simulink library "Power_FuelCell1Motor"  (R2019b)
settings: Solver=VariableStepAuto  StartTime=0.0  StopTime=10.0  RelTol=1e-3
undefined symbols (not defined in the file or in its folder): Init, Powertrain
libraries: fl_lib x84, nesl_utility x29, GasN_lib x21, SimscapeFluids_lib x6, simulink_extras x5, customMath_lib x5, ee_lib x3, gn_supplement_lib x2, simulink x2, custom_dcdc_uni_lib x1, sm_lib x1
(part 2 of 2)

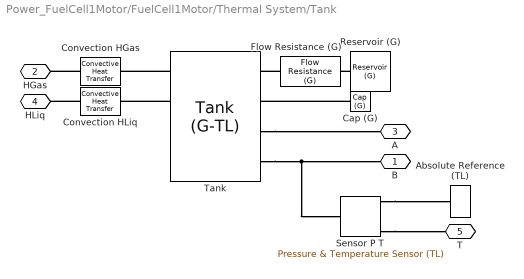
== system Power_FuelCell1Motor/FuelCell1Motor/Thermal System/Tank ==
  Absolute Reference (TL) : fl_lib/Thermal Liquid/Elements/Absolute Reference (TL)
      settings: SourceProductName=Simscape  SourceProductBaseCode=SS
  Cap (G) : fl_lib/Gas/Elements/Cap (G)  p_specify=off  p_priority=None  p=0.101325 MPa  p_nominal_specify=off  p_nominal_unit=MPa  p_nominal_value=1  T_specify=off  T_priority=None  T=293.15 K  T_nominal_specify=off  T_nominal_unit=K  T_nominal_value=1
      settings: SourceProductName=Simscape  SourceProductBaseCode=SS
  Convection HGas : fl_lib/Thermal/Thermal Elements/Convective Heat Transfer  area=1e-2 m^2  heat_tr_coeff=20 W/(m^2 * K)  T_specify=off  T_priority=None  T=0 K  T_nominal_specify=off  T_nominal_unit=K  T_nominal_value=1  Q_specify=off  Q_priority=None  Q=0 W  Q_nominal_specify=off  Q_nominal_unit=W  Q_nominal_value=1
  Convection HLiq : fl_lib/Thermal/Thermal Elements/Convective Heat Transfer  area=1e-4 m^2  heat_tr_coeff=20 W/(m^2 * K)  T_specify=off  T_priority=None  T=0 K  T_nominal_specify=off  T_nominal_unit=K  T_nominal_value=1  Q_specify=off  Q_priority=None  Q=0 W  Q_nominal_specify=off  Q_nominal_unit=W  Q_nominal_value=1
  Flow Resistance (G) : fl_lib/Gas/Elements/Flow Resistance (G)  delta_p_nominal=0.001 MPa  mdot_nominal=0.1 kg/s  rho_nominal=0 kg/m^3  area=0.01 m^2  laminar_fraction=1e-3
      settings: SourceProductName=Simscape  SourceProductBaseCode=SS  InternalSimscapePortConfiguration="{\"Bottom\":[],\"Left\":[{\"id\":\"A\",\"label\":\"A\",\"type\":\"foundation.gas.gas\"}],\"Right\":[{\"id\":\"B\",\"label\":\"B\",\"type\":\"foundation.gas.gas\"}],\"Top\":[]}"
  Reservoir (G) : fl_lib/Gas/Elements/Reservoir (G)  pressure_spec=1  reservoir_pressure=0.101325 MPa  reservoir_temperature=25 degC  area_A=0.001 m^2
      settings: SourceProductName=Simscape  SourceProductBaseCode=SS
  Sensor P T : fl_lib/Thermal Liquid/Sensors/Pressure & Temperature Sensor (TL)
      settings: SourceProductName=Simscape  SourceProductBaseCode=SS  InternalSimscapePortConfiguration="{\"Bottom\":[],\"Left\":[{\"id\":\"A\",\"label\":\"A\",\"type\":\"foundation.thermal_liquid.thermal_liquid\"}],\"Right\":[{\"id\":\"B\",\"label\":\"B\",\"type\":\"foundation.thermal_liquid.thermal_liquid\"},{\"id\":\"P\",\"label\":\"P\",\"type\":\"output\"},{\"id\":\"T\",\"label\":\"T\",\"type\":\"output\"}],\"Top\":[]}"
  Tank : SimscapeFluids_lib/Fluid Network Interfaces/Tanks & Accumulators/Tank (G-TL)  volume_total=Cooling.Tank.volume.Value m^3  volume_spec=1  tank_area=Cooling.Tank.area.Value m^2  level_TLU=[0, 3, 5] m  volume_TLU=[0, 4, 6] m^3  inlet_height=0.01 m  inlet_areas_A1B1=Cooling.Tank.areaA1B1.Value m^2  area_A2=0.01^2*pi m^2  g=9.81 m/s^2  p_gas_tank_specify=off  p_gas_tank_priority=High  p_gas_tank=0.101325 MPa  p_gas_tank_nominal_specify=off  p_gas_tank_nominal_unit=MPa  p_gas_tank_nominal_value=1  T_gas_tank_specify=on  T_gas_tank_priority=High  T_gas_tank=Cooling.Tank.TgasInit.Value K  T_gas_tank_nominal_specify=off  T_gas_tank_nominal_unit=K  T_gas_tank_nominal_value=1  rho_gas_tank_specify=off  rho_gas_tank_priority=None  rho_gas_tank=1.2 kg/m^3  rho_gas_tank_nominal_specify=off  rho_gas_tank_nominal_unit=kg/m^3  rho_gas_tank_nominal_value=1  T_liquid_tank_specify=on  T_liquid_tank_priority=High  T_liquid_tank=Cooling.Tank.TliquidInit.Value K  T_liquid_tank_nominal_specify=off  T_liquid_tank_nominal_unit=K  T_liquid_tank_nominal_value=1  level_specify=on  level_priority=High  level="Cooling.Tank.heightInit.Value  m"  level_nominal_specify=off  level_nominal_unit=m  level_nominal_value=1  volume_liquid_specify=off  volume_liquid_priority=None  volume_liquid=5 m^3  volume_liquid_nominal_specify=off  volume_liquid_nominal_unit=m^3  volume_liquid_nominal_value=1  mass_liquid_specify=off  mass_liquid_priority=None  mass_liquid=5e+3 kg  mass_liquid_nominal_specify=off  mass_liquid_nominal_unit=kg  mass_liquid_nominal_value=1  inlet_heights_A2B2=Cooling.Tank.heightA2B2.Value m  inlet_areas_A2B2=Cooling.Tank.areaA2B2.Value m^2  inlet_heights_A2B2C2=[.1, .05, 0] m  inlet_areas_A2B2C2=[.01, .01, .01] m^2
      settings: SourceProductName=Simscape Fluids  SourceProductBaseCode=SH  InternalSimscapePortConfiguration="{\"Bottom\":[],\"Left\":[{\"id\":\"A1\",\"label\":\"A1\",\"type\":\"foundation.gas.gas\"},{\"id\":\"B1\",\"label\":\"B1\",\"type\":\"foundation.gas.gas\"},{\"id\":\"A2\",\"label\":\"A2\",\"type\":\"foundation.thermal_liquid.thermal_liquid\"},{\"id\":\"B2\",\"label\":\"B2\",\"type\":\"foundation.thermal_liquid.thermal_liquid\"}],\"Right\":[{\"id\":\"H1\",\"label\":\"H1\",\"type\":\"foundation.thermal.thermal\"},{\"id\":\"H2\",\"label\":\"H2\",\"type\":\"foundation.thermal.thermal\"},{\"id\":\"V_out\",\"label\":\"V\",\"type\":\"output\"},{\"id\":\"L_out\",\"label\":\"L\",\"type\":\"output\"}],\"Top\":[]}"
  B : PMIOPort  Side=Left
  HGas : PMIOPort  Port=2  Side=Left
  A : PMIOPort  Port=3  Side=Right
  HLiq : PMIOPort  Port=4  Side=Left
  T : PMIOPort  Port=5  Side=Right
  connections:
  Flow Resistance (G)/RConn1 -- Tank/LConn1
  Tank/LConn3 -- A/RConn1
  Tank/RConn2 -- Convection HLiq/LConn1
  Reservoir (G)/LConn1 -- Flow Resistance (G)/LConn1
  Convection HGas/RConn1 -- HGas/RConn1
  Cap (G)/LConn1 -- Tank/LConn2
  Tank/LConn4 -- Sensor P T/LConn1 -- B/RConn1
  Sensor P T/RConn1 -- Absolute Reference (TL)/LConn1
  Sensor P T/RConn3 -- T/RConn1
  Convection HLiq/RConn1 -- HLiq/RConn1
  Tank/RConn1 -- Convection HGas/LConn1

== system Power_FuelCell1Motor/FuelCell1Motor/Thermal System/Thermal Circuit Converter FC ==
  Conductive Heat Transfer : fl_lib/Thermal/Thermal Elements/Conductive Heat Transfer  area=Cooling.Converter.conductionArea.Value m^2  thickness=Cooling.Converter.conductionThickness.Value m  th_cond=Cooling.Converter.conductivity.Value W/(m*K)  T_specify=off  T_priority=None  T=0 K  T_nominal_specify=off  T_nominal_unit=K  T_nominal_value=1  Q_specify=off  Q_priority=None  Q=0 W  Q_nominal_specify=off  Q_nominal_unit=W  Q_nominal_value=1
      settings: SourceProductName=Simscape
  Thermal Mass : fl_lib/Thermal/Thermal Elements/Thermal Mass  mass=Cooling.Converter.mThermal.Value kg  sp_heat=Cooling.Converter.Cp.Value J/kg/K  T_specify=off  T_priority=High  T=300 K  T_nominal_specify=off  T_nominal_unit=K  T_nominal_value=1  Q_specify=off  Q_priority=None  Q=0 W  Q_nominal_specify=off  Q_nominal_unit=W  Q_nominal_value=1
  A : PMIOPort  Side=Left
  B : PMIOPort  Port=2  Side=Right
  connections:
  Conductive Heat Transfer/RConn1 -- Thermal Mass/LConn1 -- B/RConn1
  Conductive Heat Transfer/LConn1 -- A/RConn1

== system Power_FuelCell1Motor/FuelCell1Motor/Thermal System/Thermal Circuit MotorF ==
  Case-Ambient Insulated : fl_lib/Thermal/Thermal Elements/Perfect Insulator  T_specify=off  T_priority=None  T=0 K  T_nominal_specify=off  T_nominal_unit=K  T_nominal_value=1
      settings: SourceProductName=Simscape
  Iron Stack-Case Conductance : fl_lib/Thermal/Thermal Elements/Conductive Heat Transfer  area=Cooling.MotorF.statorArea.Value cm^2  thickness=Cooling.MotorF.statorThickness.Value cm  th_cond=Cooling.MotorF.statorConductivity.Value W/(m*K)  T_specify=off  T_priority=None  T=0 K  T_nominal_specify=off  T_nominal_unit=K  T_nominal_value=1  Q_specify=off  Q_priority=None  Q=0 W  Q_nominal_specify=off  Q_nominal_unit=W  Q_nominal_value=1
      settings: SourceProductName=Simscape
  Motor Case Thermal Mass : fl_lib/Thermal/Thermal Elements/Thermal Mass  mass=Cooling.MotorF.statormThermal.Value kg  sp_heat="Cooling.MotorF.statorCp.Value  J/kg/K"  T_specify=off  T_priority=High  T=300 K  T_nominal_specify=off  T_nominal_unit=K  T_nominal_value=1  Q_specify=off  Q_priority=None  Q=0 W  Q_nominal_specify=off  Q_nominal_unit=W  Q_nominal_value=1
  Stator Iron Thermal Mass : fl_lib/Thermal/Thermal Elements/Thermal Mass  mass=Cooling.MotorF.w2smThermal.Value kg  sp_heat=Cooling.MotorF.w2sCp.Value J/kg/K  T_specify=off  T_priority=High  T=300 K  T_nominal_specify=off  T_nominal_unit=K  T_nominal_value=1  Q_specify=off  Q_priority=None  Q=0 W  Q_nominal_specify=off  Q_nominal_unit=W  Q_nominal_value=1
  Winding Conductance : fl_lib/Thermal/Thermal Elements/Conductive Heat Transfer  area=Cooling.MotorF.windingArea.Value cm^2  thickness=Cooling.MotorF.windingThickness.Value cm  th_cond=Cooling.MotorF.windingConductivity.Value W/(m*K)  T_specify=off  T_priority=None  T=0 K  T_nominal_specify=off  T_nominal_unit=K  T_nominal_value=1  Q_specify=off  Q_priority=None  Q=0 W  Q_nominal_specify=off  Q_nominal_unit=W  Q_nominal_value=1
      settings: SourceProductName=Simscape
  Winding Thermal Mass : fl_lib/Thermal/Thermal Elements/Thermal Mass  mass=Cooling.MotorF.windingmThermal.Value kg  sp_heat=Cooling.MotorF.Cp.Value J/kg/K  T_specify=off  T_priority=High  T=300 K  T_nominal_specify=off  T_nominal_unit=K  T_nominal_value=1  Q_specify=off  Q_priority=None  Q=0 W  Q_nominal_specify=off  Q_nominal_unit=W  Q_nominal_value=1
  Winding-Iron Conductance : fl_lib/Thermal/Thermal Elements/Conductive Heat Transfer  area=Cooling.MotorF.w2sArea.Value cm^2  thickness=Cooling.MotorF.w2sThickness.Value cm  th_cond=Cooling.MotorF.w2sConductivity.Value W/(m*K)  T_specify=off  T_priority=None  T=0 K  T_nominal_specify=off  T_nominal_unit=K  T_nominal_value=1  Q_specify=off  Q_priority=None  Q=0 W  Q_nominal_specify=off  Q_nominal_unit=W  Q_nominal_value=1
      settings: SourceProductName=Simscape
  A : PMIOPort  Side=Left
  B : PMIOPort  Port=2  Side=Right
  connections:
  Winding Conductance/RConn1 -- A/RConn1
  B/RConn1 -- Winding-Iron Conductance/LConn1 -- Iron Stack-Case Conductance/LConn1 -- Stator Iron Thermal Mass/LConn1
  Case-Ambient Insulated/LConn1 -- Iron Stack-Case Conductance/RConn1 -- Motor Case Thermal Mass/LConn1
  Winding Thermal Mass/LConn1 -- Winding-Iron Conductance/RConn1 -- Winding Conductance/LConn1

== system Power_FuelCell1Motor/FuelCell1Motor/Fuel Cell/Fuel Cell/Cap ==
  Absolute Reference (N Gas) : GasN_lib/Absolute Reference (N Gas)
      settings: InternalSimscapePortConfiguration="{\"Bottom\":[],\"Left\":[{\"id\":\"A\",\"label\":\"\",\"type\":\"GasN.GasN\"}],\"Right\":[],\"Top\":[]}"
  Sensor P T : GasN_lib/Pressure and Temperature Sensor (N Gas)
      settings: InternalSimscapePortConfiguration="{\"Bottom\":[],\"Left\":[{\"id\":\"A\",\"label\":\"A\",\"type\":\"GasN.GasN\"}],\"Right\":[{\"id\":\"p\",\"label\":\"p\",\"type\":\"output\"},{\"id\":\"T\",\"label\":\"T\",\"type\":\"output\"},{\"id\":\"B\",\"label\":\"B\",\"type\":\"GasN.GasN\"}],\"Top\":[]}"
  A : PMIOPort  Side=Left
  connections:
  Sensor P T/LConn1 -- A/RConn1
  Absolute Reference (N Gas)/LConn1 -- Sensor P T/RConn3

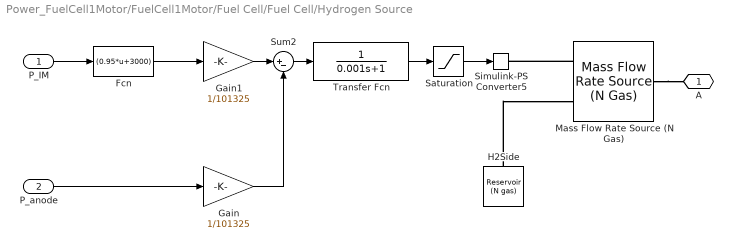
== system Power_FuelCell1Motor/FuelCell1Motor/Fuel Cell/Fuel Cell/Hydrogen Source ==
  P_IM : Inport
  P_anode : Inport  Port=2
  Fcn : Fcn  Expr=(0.95*u+3000)
  Gain : Gain  Gain=1/101325
  Gain1 : Gain  Gain=1/101325
  H2Side : GasN_lib/Reservoir (N gas)  p0=FuelCell.AnodeReservoir.p.Value MPa  T0=FuelCell.AnodeReservoir.T.Value degC  constCond=true  comp=GasN.composition_enum.mole  y0=FuelCell.AnodeReservoir.rMoleFractions.Value'  x0=[1; 0; 0; 0]  area=FuelCell.AnodeReservoir.areaPort.Value cm^2
      settings: InternalSimscapePortConfiguration="{\"Bottom\":[],\"Left\":[{\"id\":\"A\",\"label\":\"A\",\"type\":\"GasN.GasN\"}],\"Right\":[],\"Top\":[]}"
  Mass Flow Rate Source (N Gas) : GasN_lib/Mass Flow Rate Source (N Gas)  const_flow=false  flow_rate=0 kg/s  power_spec=foundation.enum.power_spec.none  area_A=FuelCell.Anode.areaPort.Value cm^2  area_B=FuelCell.Anode.areaPort.Value cm^2  mdot_A_specify=off  mdot_A_priority=None  mdot_A=0.1 kg/s  mdot_A_nominal_specify=off  mdot_A_nominal_unit=kg/s  mdot_A_nominal_value=1  mdot_B_specify=off  mdot_B_priority=None  mdot_B=0.1 kg/s  mdot_B_nominal_specify=off  mdot_B_nominal_unit=kg/s  mdot_B_nominal_value=1  phi_A_specify=off  phi_A_priority=None  phi_A=0 J/s  phi_A_nominal_specify=off  phi_A_nominal_unit=J/s  phi_A_nominal_value=1  phi_B_specify=off  phi_B_priority=None  phi_B=0 J/s  phi_B_nominal_specify=off  phi_B_nominal_unit=J/s  phi_B_nominal_value=1  mdot_A_i_specify=off  mdot_A_i_priority=None  mdot_A_i=[ 0; 0; 0; 0 ] kg/s  mdot_A_i_nominal_specify=off  mdot_A_i_nominal_unit=kg/s  mdot_A_i_nominal_value=1  mdot_B_i_specify=off  mdot_B_i_priority=None  mdot_B_i=[ 0; 0; 0; 0 ] kg/s  mdot_B_i_nominal_specify=off  mdot_B_i_nominal_unit=kg/s  mdot_B_i_nominal_value=1
      settings: InternalSimscapePortConfiguration="{\"Bottom\":[],\"Left\":[{\"id\":\"M\",\"label\":\"M\",\"type\":\"input\"},{\"id\":\"A\",\"label\":\"A\",\"type\":\"GasN.GasN\"}],\"Right\":[{\"id\":\"B\",\"label\":\"B\",\"type\":\"GasN.GasN\"}],\"Top\":[]}"
  Saturation : Saturate  UpperLimit=.1  LowerLimit=0.000001  ZeroCross=off
  Simulink-PS Converter5 : nesl_utility/Simulink-PS Converter  PhysicalDomain=network_engine_domain  SubClassName=ps_input  LeftPortType=input  RightPortType=output  PseudoPeriodic=off  Frequencies=[]  NoiseDistribution=none  NoiseParameters=[]  Unit=kg/s  AffineConversion=off  FilteringAndDerivatives=provide  SimscapeFilterOrder=1  InputFilterTimeConstant=0.001  UdotUserProvided=0
  Sum2 : Sum  Inputs=|+-  SaturateOnIntegerOverflow=on  InputSameDT=on  OutDataTypeStr=Inherit: Same as first input
  Transfer Fcn : TransferFcn  Denominator=[0.001 1]
  A : PMIOPort  Side=Right
  wires:
  Transfer Fcn/1 -> Saturation/1
  Gain1/1 -> Sum2/1
  Fcn/1 -> Gain1/1
  Saturation/1 -> Simulink-PS Converter5/1
  Gain/1 -> Sum2/2
  Sum2/1 -> Transfer Fcn/1
  P_IM/1 -> Fcn/1
  P_anode/1 -> Gain/1
  connections:
  Mass Flow Rate Source (N Gas)/LConn1 -- Simulink-PS Converter5/RConn1
  Mass Flow Rate Source (N Gas)/RConn1 -- A/RConn1
  H2Side/LConn1 -- Mass Flow Rate Source (N Gas)/LConn2

== system Power_FuelCell1Motor/FuelCell1Motor/Fuel Cell/Fuel Cell/Oxygen Source ==
  Icmd : Inport
  Chiller : Subsystem
  Compressor : Subsystem
  Desired RH : Constant  Value=FuelCell.Humidifier.relativeHdes.Value
  Gain : Gain  Gain=1.1
  Humidifier : Subsystem
  Saturation : Saturate  UpperLimit=inf  LowerLimit=0  ZeroCross=off
  B : PMIOPort  Side=Left
  P_LV : PMIOPort  Port=2  Side=Right
  N_LV : PMIOPort  Port=3  Side=Right
  pT : Outport
  Pm : Outport  Port=2
  wires:
  Saturation/1 -> Compressor/1(V)
  Compressor/2(Pm) -> Pm/1
  Gain/1 -> Saturation/1
  Desired RH/1 -> Humidifier/1(Desired RH)
  Compressor/1(pT) -> pT/1
  Icmd/1 -> Gain/1
  connections:
  Chiller/LConn1 -- Compressor/LConn1
  Humidifier/LConn1 -- Chiller/RConn1
  Compressor/RConn1 -- P_LV/RConn1
  B/RConn1 -- Humidifier/RConn1
  Compressor/RConn2 -- N_LV/RConn1

== system Power_FuelCell1Motor/FuelCell1Motor/Fuel Cell/Fuel Cell/PowerCalc ==
  PCool : Inport
  FCcurr : Inport  Port=2
  VStack : Inport  Port=3
  Pm : Inport  Port=4
  Product : Product
  Subtract : Sum  Inputs=+--
  Subtract1 : Sum
  Transfer Fcn (with initial outputs) : simulink_extras/Additional Linear/Transfer Fcn (with initial outputs)  N=[1]  D="[1  1]"  Y0=.5  U0=0
  Transfer Fcn (with initial outputs)1 : simulink_extras/Additional Linear/Transfer Fcn (with initial outputs)  N=[1]  D="[.1  1]"  Y0=0  U0=0
  Transfer Fcn (with initial outputs)2 : simulink_extras/Additional Linear/Transfer Fcn (with initial outputs)  N=[1]  D="[.1  1]"  Y0=0  U0=0
  Power : Outport
  PowerBatt : Outport  Port=2
  wires:
  PCool/1 -> Transfer Fcn (with initial outputs)1/1
  Subtract/1 -> Power/1
  VStack/1 -> Product/1
  Transfer Fcn (with initial outputs)2/1 -> Subtract/1
  FCcurr/1 -> Product/2
  Pm/1 -> Transfer Fcn (with initial outputs)/1
  Transfer Fcn (with initial outputs)1/1 -> Subtract/3, Subtract1/2
  Subtract1/1 -> PowerBatt/1
  Transfer Fcn (with initial outputs)/1 -> Subtract1/1, Subtract/2
  Product/1 -> Transfer Fcn (with initial outputs)2/1  "FCpwr"

== system Power_FuelCell1Motor/FuelCell1Motor/Fuel Cell/Fuel Cell/Sensor VI ==
  Current Sensor : fl_lib/Electrical/Electrical Sensors/Current Sensor
  Mux : Mux  Inputs=2
  PS-Simulink Converter2 : nesl_utility/PS-Simulink Converter  PhysicalDomain=network_engine_domain  SubClassName=ps_output  LeftPortType=input  RightPortType=output  PseudoPeriodic=off  Frequencies=[]  Unit=1  AffineConversion=off
  PS-Simulink Converter4 : nesl_utility/PS-Simulink Converter  PhysicalDomain=network_engine_domain  SubClassName=ps_output  LeftPortType=input  RightPortType=output  PseudoPeriodic=off  Frequencies=[]  Unit=1  AffineConversion=off
  Transfer Fcn1 : TransferFcn  Denominator=[.001 1]
  Transfer Fcn5 : TransferFcn  Denominator=[.001 1]
  Voltage Sensor2 : fl_lib/Electrical/Electrical Sensors/Voltage Sensor
  + : PMIOPort  Side=Left
  - : PMIOPort  Port=2  Side=Right
  G : PMIOPort  Port=3  Side=Right
  vi : Outport
  wires:
  PS-Simulink Converter4/1 -> Transfer Fcn5/1
  PS-Simulink Converter2/1 -> Transfer Fcn1/1
  Transfer Fcn1/1 -> Mux/2  "FCcurr"
  Transfer Fcn5/1 -> Mux/1  "FCV"
  Mux/1 -> vi/1
  connections:
  +/RConn1 -- Current Sensor/LConn1 -- Voltage Sensor2/LConn1
  PS-Simulink Converter4/LConn1 -- Voltage Sensor2/RConn1
  Current Sensor/RConn2 -- -/RConn1
  Voltage Sensor2/RConn2 -- G/RConn1
  Current Sensor/RConn1 -- PS-Simulink Converter2/LConn1

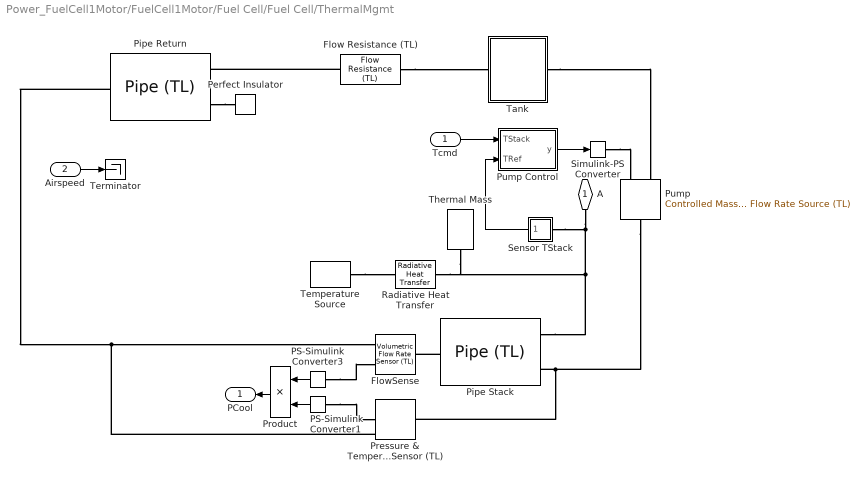
== system Power_FuelCell1Motor/FuelCell1Motor/Fuel Cell/Fuel Cell/ThermalMgmt ==
  Tcmd : Inport
  Airspeed : Inport  Port=2
  Flow Resistance (TL) : fl_lib/Thermal Liquid/Elements/Flow Resistance (TL)  delta_p_nominal=FuelCell.Thermal.Restriction.pDrop.Value MPa  mdot_nominal=FuelCell.Thermal.Restriction.mdotNominal.Value kg/s  area=FuelCell.Thermal.Restriction.areaPorts.Value m^2  laminar_fraction=FuelCell.Thermal.Restriction.rmdotLaminar.Value
      settings: SourceProductName=Simscape  SourceProductBaseCode=SS
  FlowSense : fl_lib/Thermal Liquid/Sensors/Volumetric Flow Rate Sensor (TL)
      settings: SourceProductName=Simscape  SourceProductBaseCode=SS  InternalSimscapePortConfiguration="{\"Bottom\":[],\"Left\":[{\"id\":\"A\",\"label\":\"A\",\"type\":\"foundation.thermal_liquid.thermal_liquid\"}],\"Right\":[{\"id\":\"B\",\"label\":\"B\",\"type\":\"foundation.thermal_liquid.thermal_liquid\"},{\"id\":\"V\",\"label\":\"V\",\"type\":\"output\"}],\"Top\":[]}"
  PS-Simulink Converter1 : nesl_utility/PS-Simulink Converter  PhysicalDomain=network_engine_domain  SubClassName=ps_output  LeftPortType=input  RightPortType=output  PseudoPeriodic=off  Frequencies=[]  Unit=1  AffineConversion=off
  PS-Simulink Converter3 : nesl_utility/PS-Simulink Converter  PhysicalDomain=network_engine_domain  SubClassName=ps_output  LeftPortType=input  RightPortType=output  PseudoPeriodic=off  Frequencies=[]  Unit=1  AffineConversion=off
  Perfect Insulator : fl_lib/Thermal/Thermal Elements/Perfect Insulator  T_specify=off  T_priority=None  T=0 K  T_nominal_specify=off  T_nominal_unit=K  T_nominal_value=1
      settings: SourceProductName=Simscape
  Pipe Return : fl_lib/Thermal Liquid/Elements/Pipe (TL)  length=FuelCell.Thermal.Return.pipeLength.Value cm  area=FuelCell.Thermal.Return.pipeArea.Value cm^2  Dh=FuelCell.Thermal.Return.dHydraulic.Value cm  length_add=FuelCell.Thermal.Return.xFriction.Value m  roughness=FuelCell.Thermal.Return.roughness.Value m  Re_lam=FuelCell.Thermal.Return.laminarReynoldsMax.Value  Re_tur=FuelCell.Thermal.Return.turbulentReynoldsMin.Value  shape_factor=FuelCell.Thermal.Return.frictionDarcy.Value  Nu_lam=FuelCell.Thermal.Return.laminarNusselt.Value  dynamic_compressibility=1  inertia=0  p0=FuelCell.Thermal.Return.p.Value MPa  T0=FuelCell.Thermal.Return.T.Value degC  mdot0=0 kg/s
      settings: SourceProductName=Simscape  SourceProductBaseCode=SS
  Pipe Stack : fl_lib/Thermal Liquid/Elements/Pipe (TL)  length=FuelCell.Thermal.FCStack.pipeLength.Value cm  area=FuelCell.Thermal.FCStack.pipeArea.Value cm^2  Dh=FuelCell.Thermal.FCStack.dHydraulic.Value cm  length_add=FuelCell.Thermal.FCStack.xFriction.Value m  roughness=FuelCell.Thermal.FCStack.roughness.Value m  Re_lam=FuelCell.Thermal.FCStack.laminarReynoldsMax.Value  Re_tur=FuelCell.Thermal.FCStack.turbulentReynoldsMin.Value  shape_factor=FuelCell.Thermal.FCStack.frictionDarcy.Value  Nu_lam=FuelCell.Thermal.FCStack.laminarNusselt.Value  dynamic_compressibility=simscape.enum.onoff.on  inertia=simscape.enum.onoff.off  p0="FuelCell.Thermal.FCStack.p.Value  MPa"  T0=FuelCell.Thermal.FCStack.T.Value degC  mdot0=0 kg/s
      settings: SourceProductName=Simscape  SourceProductBaseCode=SS
  Pressure & Temperature Sensor (TL) : fl_lib/Thermal Liquid/Sensors/Pressure & Temperature Sensor (TL)
      settings: SourceProductName=Simscape  SourceProductBaseCode=SS  InternalSimscapePortConfiguration="{\"Bottom\":[],\"Left\":[{\"id\":\"A\",\"label\":\"A\",\"type\":\"foundation.thermal_liquid.thermal_liquid\"}],\"Right\":[{\"id\":\"B\",\"label\":\"B\",\"type\":\"foundation.thermal_liquid.thermal_liquid\"},{\"id\":\"P\",\"label\":\"P\",\"type\":\"output\"},{\"id\":\"T\",\"label\":\"T\",\"type\":\"output\"}],\"Top\":[]}"
  Product : Product
  Pump : fl_lib/Thermal Liquid/Sources/Controlled Mass Flow Rate Source (TL)  area=FuelCell.Thermal.Pump.areaPorts.Value cm^2
      settings: SourceProductName=Simscape  SourceProductBaseCode=SS  InternalSimscapePortConfiguration="{\"Bottom\":[],\"Left\":[{\"id\":\"A\",\"label\":\"A\",\"type\":\"foundation.thermal_liquid.thermal_liquid\"},{\"id\":\"M\",\"label\":\"M\",\"type\":\"input\"}],\"Right\":[{\"id\":\"B\",\"label\":\"B\",\"type\":\"foundation.thermal_liquid.thermal_liquid\"}],\"Top\":[]}"
  Pump Control : Subsystem
  Radiative Heat Transfer : fl_lib/Thermal/Thermal Elements/Radiative Heat Transfer  area=FuelCell.Thermal.FCStack.area.Value m^2  rad_tr_coeff=FuelCell.Thermal.FCStack.kRadiation.Value W/(m^2*K^4)  T_specify=off  T_priority=None  T=0 K  T_nominal_specify=off  T_nominal_unit=K  T_nominal_value=1  Q_specify=off  Q_priority=None  Q=0 W  Q_nominal_specify=off  Q_nominal_unit=W  Q_nominal_value=1
      settings: SourceProductName=Simscape  SourceProductBaseCode=SS  InternalSimscapePortConfiguration="{\"Bottom\":[],\"Left\":[{\"id\":\"A\",\"label\":\"A\",\"type\":\"foundation.thermal.thermal\"}],\"Right\":[{\"id\":\"B\",\"label\":\"B\",\"type\":\"foundation.thermal.thermal\"}],\"Top\":[]}"
  Sensor TStack : Subsystem
  Simulink-PS Converter : nesl_utility/Simulink-PS Converter  PhysicalDomain=network_engine_domain  SubClassName=ps_input  LeftPortType=input  RightPortType=output  PseudoPeriodic=off  Frequencies=[]  NoiseDistribution=none  NoiseParameters=[]  Unit=kg/s  AffineConversion=off  FilteringAndDerivatives=filter  SimscapeFilterOrder=1  InputFilterTimeConstant=1  UdotUserProvided=0
  Tank : Subsystem
  Temperature Source : fl_lib/Thermal/Thermal Sources/Temperature Source  temperature=FuelCell.Thermal.FCStack.Tambient.Value K
      settings: SourceProductName=Simscape
  Terminator : Terminator
  Thermal Mass : fl_lib/Thermal/Thermal Elements/Thermal Mass  mass=FuelCell.Thermal.FCStack.mThermal.Value kg  sp_heat=FuelCell.Thermal.FCStack.Cp.Value J/kg/K  T_specify=on  T_priority=High  T=353.15 K  T_nominal_specify=off  T_nominal_unit=K  T_nominal_value=1  Q_specify=off  Q_priority=None  Q=0 W  Q_nominal_specify=off  Q_nominal_unit=W  Q_nominal_value=1
  A : PMIOPort  Side=Left
  PCool : Outport
  wires:
  Product/1 -> PCool/1
  Airspeed/1 -> Terminator/1
  Tcmd/1 -> Pump Control/1(TStack)
  Pump Control/1(y) -> Simulink-PS Converter/1
  Sensor TStack/1(T) -> Pump Control/2(TRef)
  PS-Simulink Converter1/1 -> Product/2
  PS-Simulink Converter3/1 -> Product/1
  connections:
  A/RConn1 -- Thermal Mass/LConn1 -- Radiative Heat Transfer/LConn1 -- Pipe Stack/LConn2 -- Sensor TStack/LConn1
  Pipe Stack/RConn1 -- FlowSense/LConn1
  PS-Simulink Converter1/LConn1 -- Pressure & Temperature Sensor (TL)/RConn2
  PS-Simulink Converter3/LConn1 -- FlowSense/RConn2
  Simulink-PS Converter/RConn1 -- Pump/LConn2
  Pressure & Temperature Sensor (TL)/RConn1 -- FlowSense/RConn1 -- Pipe Return/RConn1
  Flow Resistance (TL)/RConn1 -- Pipe Return/LConn1
  Tank/RConn1 -- Pump/LConn1
  Flow Resistance (TL)/LConn1 -- Tank/LConn1
  Pipe Return/LConn2 -- Perfect Insulator/LConn1
  Pipe Stack/LConn1 -- Pressure & Temperature Sensor (TL)/LConn1 -- Pump/RConn1
  Temperature Source/LConn1 -- Radiative Heat Transfer/RConn1

== system Power_FuelCell1Motor/FuelCell1Motor/Fuel Cell/Fuel Cell/Oxygen Source/Chiller ==
  Heat Control : Subsystem
  Heat Flow Rate Source : fl_lib/Thermal/Thermal Sources/Controlled Heat Flow Rate Source
      settings: SourceProductName=Simscape
  Pipe : GasN_lib/Pipe (N Gas)  length=FuelCell.Chiller.xPipe.Value m  area=FuelCell.Chiller.areaPipe.Value cm^2  Dh=FuelCell.Chiller.dHydraulic.Value cm  extra_length=FuelCell.Chiller.xFriction.Value m  roughness=FuelCell.Chiller.roughness.Value m  Re_lam=FuelCell.Chiller.laminarReynoldsMax.Value  Re_tur=FuelCell.Chiller.turbulentReynoldsMin.Value  shape_factor=FuelCell.Chiller.frictionDarcy.Value  Nu_lam=FuelCell.Chiller.laminarNusselt.Value  p0=FuelCell.Chiller.p.Value MPa  T0=FuelCell.Chiller.T.Value degC  comp=GasN.composition_enum.mole  y0=FuelCell.Chiller.rMoleFractions.Value'  x0=[1; 0; 0; 0]  tau_c=FuelCell.Chiller.timeCondensation.Value s  isCond=FuelCell.Chiller.speciesCondensed.Value'
      settings: InternalSimscapePortConfiguration="{\"Bottom\":[],\"Left\":[{\"id\":\"A\",\"label\":\"A\",\"type\":\"GasN.GasN\"},{\"id\":\"H\",\"label\":\"H\",\"type\":\"foundation.thermal.thermal\"},{\"id\":\"MIn\",\"label\":\"M_in\",\"type\":\"input\"},{\"id\":\"TIn\",\"label\":\"T_in\",\"type\":\"input\"}],\"Right\":[{\"id\":\"B\",\"label\":\"B\",\"type\":\"GasN.GasN\"}],\"Top\":[]}"
  Tdes : Constant  Value=FuelCell.Chiller.Tdesired.Value
  Thermal Reference : fl_lib/Thermal/Thermal Elements/Thermal Reference
  A : PMIOPort  Side=Left
  B : PMIOPort  Port=2  Side=Right
  wires:
  Tdes/1 -> Heat Control/1(TDes)
  connections:
  Thermal Reference/LConn1 -- Heat Flow Rate Source/RConn2
  B/RConn1 -- Pipe/RConn1
  Heat Flow Rate Source/LConn1 -- Pipe/LConn2
  Pipe/LConn1 -- Heat Control/RConn2
  A/RConn1 -- Heat Control/LConn1
  Heat Control/RConn1 -- Heat Flow Rate Source/RConn1

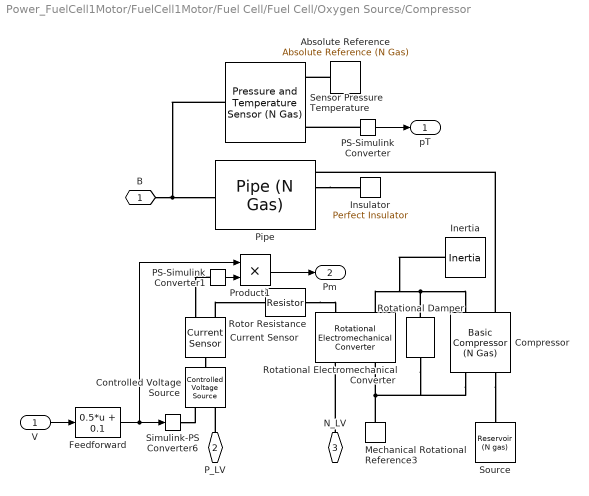
== system Power_FuelCell1Motor/FuelCell1Motor/Fuel Cell/Fuel Cell/Oxygen Source/Compressor ==
  V : Inport
  Absolute Reference : GasN_lib/Absolute Reference (N Gas)
      settings: InternalSimscapePortConfiguration="{\"Bottom\":[],\"Left\":[{\"id\":\"A\",\"label\":\"\",\"type\":\"GasN.GasN\"}],\"Right\":[],\"Top\":[]}"
  Compressor : GasN_lib/Basic Compressor (N Gas)  pr_des=FuelCell.Compressor.rPressure.Value  mdot_corr_des=FuelCell.Compressor.mdotDesign.Value kg/s  omega_corr_des=FuelCell.Compressor.wDesign.Value rad/s  p_ref=FuelCell.Compressor.pReference.Value MPa  T_ref=FuelCell.Compressor.TReference.Value K  RH_ref=FuelCell.Compressor.relHumidity.Value  b1=FuelCell.Compressor.kSpeedCurve.Value  b2=FuelCell.Compressor.kSpeedOffset.Value  b3=FuelCell.Compressor.kSpeedSharp.Value  eta_poly=FuelCell.Compressor.effPolytropic.Value  eta_mech=FuelCell.Compressor.effMechanical.Value  area_A=FuelCell.Compressor.areaInlet.Value cm^2  area_B=FuelCell.Compressor.areaOutlet.Value cm^2  mdot_A_specify=off  mdot_A_priority=None  mdot_A=0.1 kg/s  mdot_A_nominal_specify=off  mdot_A_nominal_unit=kg/s  mdot_A_nominal_value=1  mdot_B_specify=off  mdot_B_priority=None  mdot_B=0.1 kg/s  mdot_B_nominal_specify=off  mdot_B_nominal_unit=kg/s  mdot_B_nominal_value=1  Phi_A_specify=off  Phi_A_priority=None  Phi_A=0 J/s  Phi_A_nominal_specify=off  Phi_A_nominal_unit=J/s  Phi_A_nominal_value=1  Phi_B_specify=off  Phi_B_priority=None  Phi_B=0 J/s  Phi_B_nominal_specify=off  Phi_B_nominal_unit=J/s  Phi_B_nominal_value=1  mdot_A_i_specify=off  mdot_A_i_priority=None  mdot_A_i=[ 0; 0; 0; 0 ] kg/s  mdot_A_i_nominal_specify=off  mdot_A_i_nominal_unit=kg/s  mdot_A_i_nominal_value=1  mdot_B_i_specify=off  mdot_B_i_priority=None  mdot_B_i=[ 0; 0; 0; 0 ] kg/s  mdot_B_i_nominal_specify=off  mdot_B_i_nominal_unit=kg/s  mdot_B_i_nominal_value=1  torque_specify=off  torque_priority=None  torque=1 N*m  torque_nominal_specify=off  torque_nominal_unit=N*m  torque_nominal_value=1
      settings: InternalSimscapePortConfiguration="{\"Bottom\":[],\"Left\":[{\"id\":\"A\",\"label\":\"A\",\"type\":\"GasN.GasN\"},{\"id\":\"Case\",\"label\":\"C\",\"type\":\"foundation.mechanical.rotational.rotational\"}],\"Right\":[{\"id\":\"B\",\"label\":\"B\",\"type\":\"GasN.GasN\"},{\"id\":\"Rod\",\"label\":\"R\",\"type\":\"foundation.mechanical.rotational.rotational\"}],\"Top\":[]}"
  Controlled Voltage Source : fl_lib/Electrical/Electrical Sources/Controlled Voltage Source
  Current Sensor : fl_lib/Electrical/Electrical Sensors/Current Sensor
  Feedforward : Fcn  Expr=0.5*u + 0.1
  Inertia : fl_lib/Mechanical/Rotational Elements/Inertia  inertia=FuelCell.Compressor.J.Value kg*m^2  w_specify=on  w_priority=High  w=0 rad/s  w_nominal_specify=off  w_nominal_unit=rad/s  w_nominal_value=1  t_specify=off  t_priority=None  t=0 N*m  t_nominal_specify=off  t_nominal_unit=N*m  t_nominal_value=1
  Insulator : fl_lib/Thermal/Thermal Elements/Perfect Insulator  T_specify=off  T_priority=None  T=0 K  T_nominal_specify=off  T_nominal_unit=K  T_nominal_value=1
      settings: SourceProductName=Simscape
  Mechanical Rotational Reference3 : fl_lib/Mechanical/Rotational Elements/Mechanical Rotational Reference
  PS-Simulink Converter : nesl_utility/PS-Simulink Converter  PhysicalDomain=network_engine_domain  SubClassName=ps_output  LeftPortType=input  RightPortType=output  PseudoPeriodic=off  Frequencies=[]  Unit=Pa  AffineConversion=off
  PS-Simulink Converter1 : nesl_utility/PS-Simulink Converter  PhysicalDomain=network_engine_domain  SubClassName=ps_output  LeftPortType=input  RightPortType=output  PseudoPeriodic=off  Frequencies=[]  Unit=A  AffineConversion=off
  Pipe : GasN_lib/Pipe (N Gas)  length=FuelCell.CompressorPipe.xPipe.Value m  area=FuelCell.CompressorPipe.areaPipe.Value cm^2  Dh=FuelCell.CompressorPipe.dHydraulic.Value cm  extra_length=FuelCell.CompressorPipe.xFriction.Value m  roughness=FuelCell.CompressorPipe.roughness.Value m  Re_lam=FuelCell.CompressorPipe.laminarReynoldsMax.Value  Re_tur=FuelCell.CompressorPipe.turbulentReynoldsMin.Value  shape_factor=FuelCell.CompressorPipe.frictionDarcy.Value  Nu_lam=FuelCell.CompressorPipe.laminarNusselt.Value  p0=FuelCell.CompressorPipe.p.Value MPa  T0=FuelCell.CompressorPipe.T.Value degC  comp=GasN.composition_enum.mole  y0=FuelCell.CompressorPipe.rMoleFractions.Value'  x0=[1; 0; 0; 0]  tau_c=FuelCell.CompressorPipe.timeCondensation.Value s  isCond=FuelCell.CompressorPipe.speciesCondensed.Value'
      settings: InternalSimscapePortConfiguration="{\"Bottom\":[],\"Left\":[{\"id\":\"A\",\"label\":\"A\",\"type\":\"GasN.GasN\"},{\"id\":\"H\",\"label\":\"H\",\"type\":\"foundation.thermal.thermal\"},{\"id\":\"MIn\",\"label\":\"M_in\",\"type\":\"input\"},{\"id\":\"TIn\",\"label\":\"T_in\",\"type\":\"input\"}],\"Right\":[{\"id\":\"B\",\"label\":\"B\",\"type\":\"GasN.GasN\"}],\"Top\":[]}"
  Product1 : Product
  Rotational Electromechanical Converter : fl_lib/Electrical/Electrical Elements/Rotational Electromechanical Converter  K=FuelCell.Compressor.KMotor.Value V/(rad/s)  i_specify=off  i_priority=None  i=0 A  i_nominal_specify=off  i_nominal_unit=A  i_nominal_value=1  v_specify=off  v_priority=None  v=0 V  v_nominal_specify=off  v_nominal_unit=V  v_nominal_value=1  t_specify=off  t_priority=None  t=0 N*m  t_nominal_specify=off  t_nominal_unit=N*m  t_nominal_value=1  w_specify=off  w_priority=None  w=0 rad/s  w_nominal_specify=off  w_nominal_unit=rad/s  w_nominal_value=1
      settings: SourceProductName=Simscape
  Rotational Damper : fl_lib/Mechanical/Rotational Elements/Rotational Damper  D=FuelCell.Compressor.b.Value N*m/(rad/s)  w_specify=off  w_priority=None  w=0 rad/s  w_nominal_specify=off  w_nominal_unit=rad/s  w_nominal_value=1  t_specify=off  t_priority=None  t=0 N*m  t_nominal_specify=off  t_nominal_unit=N*m  t_nominal_value=1
  Rotor Resistance : fl_lib/Electrical/Electrical Elements/Resistor  Tag=Factory Generic  R=FuelCell.Compressor.rMotor.Value Ohm  i_specify=off  i_priority=High  i=0 A  i_nominal_specify=off  i_nominal_unit=A  i_nominal_value=1  v_specify=off  v_priority=High  v=0 V  v_nominal_specify=off  v_nominal_unit=V  v_nominal_value=1
  Sensor Pressure Temperature : GasN_lib/Pressure and Temperature Sensor (N Gas)
      settings: InternalSimscapePortConfiguration="{\"Bottom\":[],\"Left\":[{\"id\":\"A\",\"label\":\"A\",\"type\":\"GasN.GasN\"}],\"Right\":[{\"id\":\"p\",\"label\":\"p\",\"type\":\"output\"},{\"id\":\"T\",\"label\":\"T\",\"type\":\"output\"},{\"id\":\"B\",\"label\":\"B\",\"type\":\"GasN.GasN\"}],\"Top\":[]}"
  Simulink-PS Converter6 : nesl_utility/Simulink-PS Converter  PhysicalDomain=network_engine_domain  SubClassName=ps_input  LeftPortType=input  RightPortType=output  PseudoPeriodic=off  Frequencies=[]  NoiseDistribution=none  NoiseParameters=[]  Unit=V  AffineConversion=off  FilteringAndDerivatives=filter  SimscapeFilterOrder=1  InputFilterTimeConstant=0.01  UdotUserProvided=0
  Source : GasN_lib/Reservoir (N gas)  p0=FuelCell.CompressorSource.p.Value MPa  T0=FuelCell.CompressorSource.T.Value degC  constCond=true  comp=GasN.composition_enum.mole  y0=FuelCell.CompressorSource.rMoleFractions.Value'  x0=[1; 0; 0; 0]  area=FuelCell.CompressorSource.areaPipe.Value cm^2
      settings: InternalSimscapePortConfiguration="{\"Bottom\":[],\"Left\":[{\"id\":\"A\",\"label\":\"A\",\"type\":\"GasN.GasN\"}],\"Right\":[],\"Top\":[]}"
  B : PMIOPort  Side=Left
  P_LV : PMIOPort  Port=2  Side=Right
  N_LV : PMIOPort  Port=3  Side=Right
  pT : Outport
  Pm : Outport  Port=2
  wires:
  V/1 -> Feedforward/1
  PS-Simulink Converter/1 -> pT/1
  Product1/1 -> Pm/1
  PS-Simulink Converter1/1 -> Product1/2
  Feedforward/1 -> Product1/1, Simulink-PS Converter6/1
  connections:
  Rotational Damper/LConn1 -- Rotational Electromechanical Converter/LConn2 -- Inertia/LConn1 -- Compressor/RConn2
  Simulink-PS Converter6/RConn1 -- Controlled Voltage Source/RConn1
  P_LV/RConn1 -- Controlled Voltage Source/RConn2
  N_LV/RConn1 -- Rotational Electromechanical Converter/RConn1
  Mechanical Rotational Reference3/LConn1 -- Compressor/LConn2 -- Rotational Damper/RConn1 -- Rotational Electromechanical Converter/RConn2
  Current Sensor/LConn1 -- Controlled Voltage Source/LConn1
  Current Sensor/RConn2 -- Rotor Resistance/LConn1
  B/RConn1 -- Sensor Pressure Temperature/LConn1 -- Pipe/RConn1
  Absolute Reference/LConn1 -- Sensor Pressure Temperature/RConn3
  PS-Simulink Converter/LConn1 -- Sensor Pressure Temperature/RConn1
  Compressor/RConn1 -- Pipe/LConn1
  Compressor/LConn1 -- Source/LConn1
  PS-Simulink Converter1/LConn1 -- Current Sensor/RConn1
  Rotor Resistance/RConn1 -- Rotational Electromechanical Converter/LConn1
  Pipe/LConn2 -- Insulator/LConn1

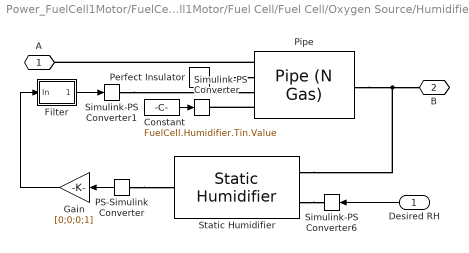
== system Power_FuelCell1Motor/FuelCell1Motor/Fuel Cell/Fuel Cell/Oxygen Source/Humidifier ==
  Desired RH : Inport
  Constant : Constant  Value=FuelCell.Humidifier.Tin.Value
  Filter : Subsystem  mask(First-order lag supporting vector signals){b=[1 1 1 1]*0.01, x_initial=[0 0 0 0]}
      mask prompts: b "Filter time constant"; x_initial "Initial output"
      mask help: Models a lag of the form 1/(b*s+1) where s is the Laplace operator.
  Gain : Gain  Gain=[0;0;0;1]
  PS-Simulink Converter : nesl_utility/PS-Simulink Converter  PhysicalDomain=network_engine_domain  SubClassName=ps_output  LeftPortType=input  RightPortType=output  PseudoPeriodic=off  Frequencies=[]  Unit=1  AffineConversion=off
  Perfect Insulator : fl_lib/Thermal/Thermal Elements/Perfect Insulator  T_specify=off  T_priority=None  T=0 K  T_nominal_specify=off  T_nominal_unit=K  T_nominal_value=1
      settings: SourceProductName=Simscape
  Pipe : GasN_lib/Pipe (N Gas)  length=FuelCell.Humidifier.xPipe.Value m  area=FuelCell.Humidifier.areaPipe.Value cm^2  Dh=FuelCell.Humidifier.dHydraulic.Value cm  extra_length=FuelCell.Humidifier.xFriction.Value m  roughness=FuelCell.Humidifier.roughness.Value m  Re_lam=FuelCell.Humidifier.laminarReynoldsMax.Value  Re_tur=FuelCell.Humidifier.turbulentReynoldsMin.Value  shape_factor=FuelCell.Humidifier.frictionDarcy.Value  Nu_lam=FuelCell.Humidifier.laminarNusselt.Value  p0=FuelCell.Humidifier.p.Value MPa  T0=FuelCell.Humidifier.T.Value degC  comp=GasN.composition_enum.mole  y0=FuelCell.Humidifier.rMoleFractions.Value'  x0=[1; 0; 0; 0]  tau_c=FuelCell.Humidifier.timeCondensation.Value s  isCond=FuelCell.Humidifier.speciesCondensed.Value'
      settings: InternalSimscapePortConfiguration="{\"Bottom\":[],\"Left\":[{\"id\":\"A\",\"label\":\"A\",\"type\":\"GasN.GasN\"},{\"id\":\"H\",\"label\":\"H\",\"type\":\"foundation.thermal.thermal\"},{\"id\":\"MIn\",\"label\":\"M_in\",\"type\":\"input\"},{\"id\":\"TIn\",\"label\":\"T_in\",\"type\":\"input\"}],\"Right\":[{\"id\":\"B\",\"label\":\"B\",\"type\":\"GasN.GasN\"}],\"Top\":[]}"
  Simulink-PS Converter : nesl_utility/Simulink-PS Converter  PhysicalDomain=network_engine_domain  SubClassName=ps_input  LeftPortType=input  RightPortType=output  PseudoPeriodic=off  Frequencies=[]  NoiseDistribution=none  NoiseParameters=[]  Unit=1  AffineConversion=off  FilteringAndDerivatives=provide  SimscapeFilterOrder=1  InputFilterTimeConstant=0.001  UdotUserProvided=0
  Simulink-PS Converter1 : nesl_utility/Simulink-PS Converter  PhysicalDomain=network_engine_domain  SubClassName=ps_input  LeftPortType=input  RightPortType=output  PseudoPeriodic=off  Frequencies=[]  NoiseDistribution=none  NoiseParameters=[]  Unit=1  AffineConversion=off  FilteringAndDerivatives=provide  SimscapeFilterOrder=1  InputFilterTimeConstant=0.001  UdotUserProvided=0
  Simulink-PS Converter6 : nesl_utility/Simulink-PS Converter  PhysicalDomain=network_engine_domain  SubClassName=ps_input  LeftPortType=input  RightPortType=output  PseudoPeriodic=off  Frequencies=[]  NoiseDistribution=none  NoiseParameters=[]  Unit=1  AffineConversion=off  FilteringAndDerivatives=provide  SimscapeFilterOrder=1  InputFilterTimeConstant=0.001  UdotUserProvided=0
  Static Humidifier : gn_supplement_lib/Static Humidifier  Kp=0.5 kg/s
      settings: InternalSimscapePortConfiguration="{\"Bottom\":[],\"Left\":[{\"id\":\"Rh_des\",\"label\":\"Rh_des\",\"type\":\"input\"},{\"id\":\"A\",\"label\":\"A\",\"type\":\"GasN.GasN\"}],\"Right\":[{\"id\":\"m_add\",\"label\":\"m_add\",\"type\":\"output\"}],\"Top\":[]}"
  A : PMIOPort  Side=Left
  B : PMIOPort  Port=2  Side=Right
  wires:
  Desired RH/1 -> Simulink-PS Converter6/1
  Constant/1 -> Simulink-PS Converter/1
  PS-Simulink Converter/1 -> Gain/1
  Gain/1 -> Filter/1(In)
  Filter/1(Out) -> Simulink-PS Converter1/1
  connections:
  Pipe/RConn1 -- Static Humidifier/LConn2 -- B/RConn1
  Pipe/LConn1 -- A/RConn1
  Static Humidifier/LConn1 -- Simulink-PS Converter6/RConn1
  PS-Simulink Converter/LConn1 -- Static Humidifier/RConn1
  Simulink-PS Converter1/RConn1 -- Pipe/LConn3
  Pipe/LConn4 -- Simulink-PS Converter/RConn1
  Perfect Insulator/LConn1 -- Pipe/LConn2

== system Power_FuelCell1Motor/FuelCell1Motor/Fuel Cell/Fuel Cell/ThermalMgmt/Pump Control ==
  TStack : Inport
  TRef : Inport  Port=2
  PID Controller : simulink/Continuous/PID Controller  Controller=PID  Form=Parallel  TimeDomain=Continuous-time  SampleTime=-1  IntegratorMethod=Forward Euler  FilterMethod=Forward Euler  ControllerParametersSource=internal  P=FuelCell.Thermal.PumpCtrl.Kp.Value  I=FuelCell.Thermal.PumpCtrl.Ki.Value  D=FuelCell.Thermal.PumpCtrl.Kd.Value  UseFilter=on  N=FuelCell.Thermal.PumpCtrl.filter.Value  TunerSelectOption=Transfer Function Based (PID Tuner App)  ZeroCross=off  InitialConditionSource=internal  InitialConditionForIntegrator=0  InitialConditionForFilter=0  DifferentiatorICPrevScaledInput=0  ExternalReset=none  TrackingMode=off  Kt=1  LimitOutput=on  UpperSaturationLimit=FuelCell.Thermal.PumpCtrl.upperlim.Value  LowerSaturationLimit=FuelCell.Thermal.PumpCtrl.lowerlim.Value  LinearizeAsGain=on  AntiWindupMode=clamping  Kb=1  POutMin=[]  POutMax=[]  IOutMin=[]  IOutMax=[]  DOutMin=[]  DOutMax=[]  NOutMin=[]  NOutMax=[]  SumOutMin=[]  SumOutMax=[]  SaturationOutMin=[]  SaturationOutMax=[]  PParamMin=[]  PParamMax=[]  IParamMin=[]  IParamMax=[]  DParamMin=[]  DParamMax=[]  NParamMin=[]  NParamMax=[]  KbParamMin=[]  KbParamMax=[]  KtParamMin=[]  KtParamMax=[]  KbOutMin=[]  KbOutMax=[]  KtOutMin=[]  KtOutMax=[]  IntegratorOutMin=[]  IntegratorOutMax=[]  FilterOutMin=[]  FilterOutMax=[]  SumI1OutMin=[]  SumI1OutMax=[]  SumI2OutMin=[]  SumI2OutMax=[]  SumI3OutMin=[]  SumI3OutMax=[]  SumI4OutMin=[]  SumI4OutMax=[]  SumDOutMin=[]  SumDOutMax=[]  DifferentiatorOutMin=[]  DifferentiatorOutMax=[]  FilterDiffOutCoefMin=[]  FilterDiffOutCoefMax=[]  ReciprocalOutMin=[]  ReciprocalOutMax=[]  SumDenOutMin=[]  SumDenOutMax=[]  SumNumOutMin=[]  SumNumOutMax=[]  DivideOutMin=[]  DivideOutMax=[]  IntegratorContinuousStateAttributes=''  IntegratorStateMustResolveToSignalObject=off  IntegratorRTWStateStorageClass=Auto  FilterContinuousStateAttributes=''  FilterStateMustResolveToSignalObject=off  FilterRTWStateStorageClass=Auto  ParallelPVariant=InternalParameters  IdealPVariant=Disabled  IVariant=InternalParameters  DVariant=InternalParameters  IntegratorVariant=Continuous  SatVariant=Enabled  AWVariant=ContClampingParallel  PCopyVariant=Disabled  TRVariant=Disabled  FdbkBlocksVariant=Forward  IdealPFdbkVariant=Disabled  SatFdbkVariant=Disabled  DerivativeFilterVariant=ContFilter  NVariant=InternalParameters  NCopyVariant=Disabled  FilterICVariant=InternalICsFilter  IntegratorICVariant=InternalICs  ExternalResetVariant=Disabled  TRSumVariant=Passthrough  SumFdbkVariant=Disabled  SumVariant=Sum_PID
  Subtract : Sum  Inputs=+-
  Transfer Fcn (with initial outputs)1 : simulink_extras/Additional Linear/Transfer Fcn (with initial outputs)  N=[1]  D="[1  1]"  Y0=.5  U0=80
  y : Outport
  wires:
  Subtract/1 -> PID Controller/1
  Transfer Fcn (with initial outputs)1/1 -> Subtract/1
  TRef/1 -> Transfer Fcn (with initial outputs)1/1
  PID Controller/1 -> y/1
  TStack/1 -> Subtract/2

== system Power_FuelCell1Motor/FuelCell1Motor/Fuel Cell/Fuel Cell/ThermalMgmt/Sensor TStack ==
  PS-Simulink Converter2 : nesl_utility/PS-Simulink Converter  PhysicalDomain=network_engine_domain  SubClassName=ps_output  LeftPortType=input  RightPortType=output  PseudoPeriodic=off  Frequencies=[]  Unit=degC  AffineConversion=on
  Temperature Sensor : fl_lib/Thermal/Thermal Sensors/Temperature Sensor
  Thermal Reference : fl_lib/Thermal/Thermal Elements/Thermal Reference
  A : PMIOPort  Side=Left
  T : Outport
  wires:
  PS-Simulink Converter2/1 -> T/1
  connections:
  Thermal Reference/LConn1 -- Temperature Sensor/RConn1
  PS-Simulink Converter2/LConn1 -- Temperature Sensor/RConn2
  Temperature Sensor/LConn1 -- A/RConn1

== system Power_FuelCell1Motor/FuelCell1Motor/Fuel Cell/Fuel Cell/ThermalMgmt/Tank ==
  Perfect Insulator : fl_lib/Thermal/Thermal Elements/Perfect Insulator  T_specify=off  T_priority=None  T=0 K  T_nominal_specify=off  T_nominal_unit=K  T_nominal_value=1
      settings: SourceProductName=Simscape
  Tank : SimscapeFluids_lib/Thermal Liquid/Tanks & Accumulators/Tank (TL)  pressure_spec=1  tank_pressure=0.101325 MPa  max_capacity=FuelCell.Thermal.Tank.volume.Value l  volume_spec=1  tank_area=FuelCell.Thermal.Tank.area.Value cm^2  level_TLU=[0, 3, 5] m  volume_TLU=[0, 4, 6] m^3  inlet_height=0.1 m  inlet_area=0.01 m^2  g=FuelCell.Thermal.Tank.g.Value m/s^2  level_specify=on  level_priority=None  level=0 m  level_nominal_specify=off  level_nominal_unit=m  level_nominal_value=1  volume_specify=on  volume_priority=High  volume=FuelCell.Thermal.Tank.volumeLiquid.Value l  volume_nominal_specify=off  volume_nominal_unit=m^3  volume_nominal_value=1  mass_specify=off  mass_priority=None  mass=5e+3 kg  mass_nominal_specify=off  mass_nominal_unit=kg  mass_nominal_value=1  T_tank_specify=off  T_tank_priority=High  T_tank=293.15 K  T_tank_nominal_specify=off  T_tank_nominal_unit=K  T_tank_nominal_value=1  inlet_heights_AB=FuelCell.Thermal.Tank.elevationAB.Value m  inlet_areas_AB=FuelCell.Thermal.Tank.areaAB.Value cm^2  inlet_heights_ABC=[.1, .05, 0] m  inlet_areas_ABC=[.01, .01, .01] m^2
      settings: SourceProductName=Simscape Fluids  SourceProductBaseCode=SH  InternalSimscapePortConfiguration="{\"Bottom\":[],\"Left\":[{\"id\":\"A\",\"label\":\"A\",\"type\":\"foundation.thermal_liquid.thermal_liquid\"},{\"id\":\"B\",\"label\":\"B\",\"type\":\"foundation.thermal_liquid.thermal_liquid\"}],\"Right\":[{\"id\":\"V_out\",\"label\":\"V\",\"type\":\"output\"},{\"id\":\"L_out\",\"label\":\"L\",\"type\":\"output\"},{\"id\":\"T_out\",\"label\":\"T\",\"type\":\"output\"},{\"id\":\"H\",\"label\":\"H\",\"type\":\"foundation.thermal.thermal\"}],\"Top\":[]}"
  A : PMIOPort  Side=Right
  B : PMIOPort  Port=2  Side=Left
  connections:
  Tank/RConn4 -- Perfect Insulator/LConn1
  Tank/LConn1 -- A/RConn1
  B/RConn1 -- Tank/LConn2

== system Power_FuelCell1Motor/FuelCell1Motor/Fuel Cell/Fuel Cell/Oxygen Source/Chiller/Heat Control ==
  TDes : Inport
  Absolute Reference (N Gas) : GasN_lib/Absolute Reference (N Gas)
      settings: InternalSimscapePortConfiguration="{\"Bottom\":[],\"Left\":[{\"id\":\"A\",\"label\":\"\",\"type\":\"GasN.GasN\"}],\"Right\":[],\"Top\":[]}"
  PS Subtract : customMath_lib/PS Subtract
      settings: InternalSimscapePortConfiguration="{\"Bottom\":[],\"Left\":[{\"id\":\"I1\",\"label\":\"\",\"type\":\"input\"},{\"id\":\"I2\",\"label\":\"\",\"type\":\"input\"}],\"Right\":[{\"id\":\"O\",\"label\":\"\",\"type\":\"output\"}],\"Top\":[]}"
  Product M cp : customMath_lib/PS Custom Product
      settings: InternalSimscapePortConfiguration="{\"Bottom\":[],\"Left\":[{\"id\":\"I1\",\"label\":\"\",\"type\":\"input\"},{\"id\":\"I2\",\"label\":\"\",\"type\":\"input\"}],\"Right\":[{\"id\":\"O\",\"label\":\"\",\"type\":\"output\"}],\"Top\":[]}"
  Product Q : customMath_lib/PS Custom Product
      settings: InternalSimscapePortConfiguration="{\"Bottom\":[],\"Left\":[{\"id\":\"I1\",\"label\":\"\",\"type\":\"input\"},{\"id\":\"I2\",\"label\":\"\",\"type\":\"input\"}],\"Right\":[{\"id\":\"O\",\"label\":\"\",\"type\":\"output\"}],\"Top\":[]}"
  Sensor Mass Flow Rate : GasN_lib/Mass Flow Rate Sensor (N Gas)
      settings: InternalSimscapePortConfiguration="{\"Bottom\":[],\"Left\":[{\"id\":\"A\",\"label\":\"A\",\"type\":\"GasN.GasN\"}],\"Right\":[{\"id\":\"M\",\"label\":\"M\",\"type\":\"output\"},{\"id\":\"Phi_out\",\"label\":\"Phi\",\"type\":\"output\"},{\"id\":\"M_i\",\"label\":\"M_i\",\"type\":\"output\"},{\"id\":\"B\",\"label\":\"B\",\"type\":\"GasN.GasN\"}],\"Top\":[]}"
  Sensor P T : GasN_lib/Pressure and Temperature Sensor (N Gas)
      settings: InternalSimscapePortConfiguration="{\"Bottom\":[],\"Left\":[{\"id\":\"A\",\"label\":\"A\",\"type\":\"GasN.GasN\"}],\"Right\":[{\"id\":\"p\",\"label\":\"p\",\"type\":\"output\"},{\"id\":\"T\",\"label\":\"T\",\"type\":\"output\"},{\"id\":\"B\",\"label\":\"B\",\"type\":\"GasN.GasN\"}],\"Top\":[]}"
  Sensor Thermo : GasN_lib/Thermodynamic Properties Sensor (N Gas)
      settings: InternalSimscapePortConfiguration="{\"Bottom\":[],\"Left\":[{\"id\":\"A\",\"label\":\"A\",\"type\":\"GasN.GasN\"}],\"Right\":[{\"id\":\"H\",\"label\":\"h\",\"type\":\"output\"},{\"id\":\"RHO\",\"label\":\"rho\",\"type\":\"output\"},{\"id\":\"CP\",\"label\":\"cp\",\"type\":\"output\"},{\"id\":\"S\",\"label\":\"s\",\"type\":\"output\"}],\"Top\":[]}"
  Simulink-PS Converter4 : nesl_utility/Simulink-PS Converter  PhysicalDomain=network_engine_domain  SubClassName=ps_input  LeftPortType=input  RightPortType=output  PseudoPeriodic=off  Frequencies=[]  NoiseDistribution=none  NoiseParameters=[]  Unit=K  AffineConversion=off  FilteringAndDerivatives=provide  SimscapeFilterOrder=1  InputFilterTimeConstant=0.001  UdotUserProvided=0
  A : PMIOPort  Side=Left
  Q : PMIOPort  Port=2  Side=Right
  B : PMIOPort  Port=3  Side=Right
  wires:
  TDes/1 -> Simulink-PS Converter4/1
  connections:
  Sensor P T/LConn1 -- Sensor Thermo/LConn1 -- A/RConn1 -- Sensor Mass Flow Rate/LConn1
  Product M cp/LConn2 -- Sensor Thermo/RConn3
  PS Subtract/LConn2 -- Sensor P T/RConn2
  Product M cp/LConn1 -- Sensor Mass Flow Rate/RConn1
  PS Subtract/RConn1 -- Product Q/LConn2
  Product M cp/RConn1 -- Product Q/LConn1
  Absolute Reference (N Gas)/LConn1 -- Sensor P T/RConn3
  PS Subtract/LConn1 -- Simulink-PS Converter4/RConn1
  Product Q/RConn1 -- Q/RConn1
  B/RConn1 -- Sensor Mass Flow Rate/RConn4

== system Power_FuelCell1Motor/FuelCell1Motor/Fuel Cell/Fuel Cell/Oxygen Source/Humidifier/Filter ==
  In : Inport
  Gain : Gain  Gain=1./b
  Integrator : Integrator  InitialCondition=x_initial.*b
  Sum : Sum  Inputs=|+-  SaturateOnIntegerOverflow=on  InputSameDT=on  OutDataTypeStr=Inherit: Same as first input
  Out : Outport  VectorParamsAs1DForOutWhenUnconnected=off
  wires:
  Gain/1 -> Out/1, Sum/2
  Integrator/1 -> Gain/1
  In/1 -> Sum/1
  Sum/1 -> Integrator/1
